simulink model "SineWaves"  (R2024a)
settings: Solver=VariableStepAuto  StartTime=0.0  StopTime=10.0  MaxStep=0.01  RelTol=1e-3
settings Model: Creator=ammaa  LastModifiedBy=ammaa

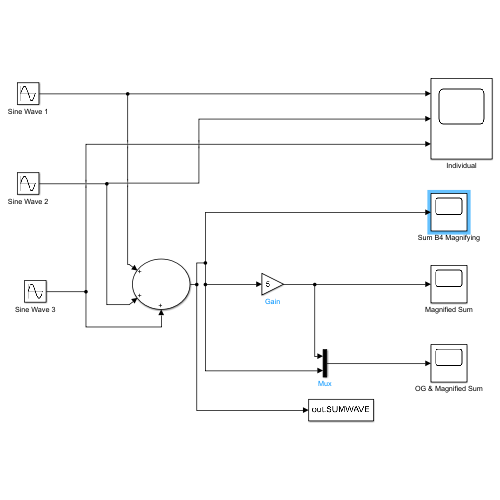
[thumbnail: Simulink's stored preview of the top-level diagram]
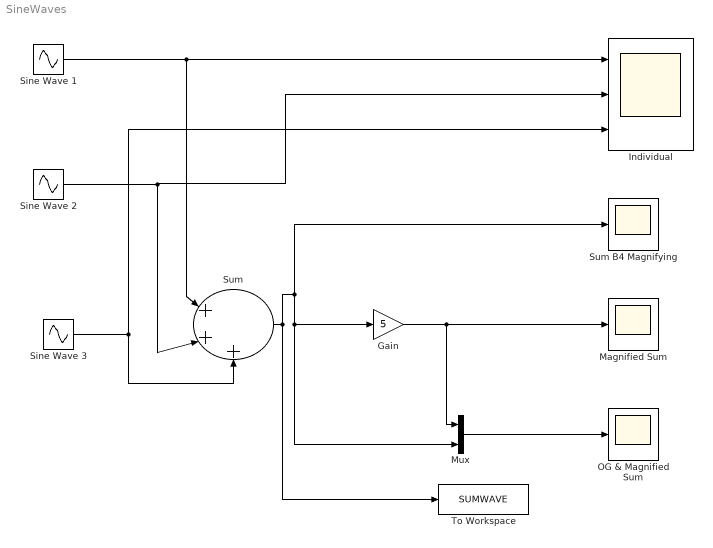
== system SineWaves ==
  Gain : Gain  Gain=5
  Individual : Scope  NumInputPorts=3
  Magnified Sum : Scope
  Mux : Mux  Inputs=2
  OG & Magnified Sum : Scope
  Sine Wave 1 : Sin  SampleTime=0
  Sine Wave 2 : Sin  Frequency=5  SampleTime=0
  Sine Wave 3 : Sin  Frequency=10  SampleTime=0
  Sum : Sum  Inputs=|+++
  Sum B4 Magnifying : Scope
  To Workspace : ToWorkspace  VariableName=SUMWAVE  SaveFormat=Timeseries  SampleTime=-1
  wires:
  Sine Wave 1/1 -> Sum/1, Individual/1
  Sine Wave 2/1 -> Sum/2, Individual/2
  Sine Wave 3/1 -> Sum/3, Individual/3
  Sum/1 -> Mux/2, Gain/1, Sum B4 Magnifying/1, To Workspace/1
  Gain/1 -> Mux/1, Magnified Sum/1
  Mux/1 -> OG & Magnified Sum/1
